simulink model "Simulink_Model_by_NV_PATEL"  (R2022a)
settings: Solver=VariableStepAuto  StartTime=0.0  StopTime=15  FixedStep=0.01  RelTol=1e-3
values from neighbouring files (symbols this model uses):
  direct_transmission_matrix = 0    [state_space_and_other_parameters.m]
  input_matrix = [0; 1/(m*l^2)]    [state_space_and_other_parameters.m]
  output_matrix = [1 0]    [state_space_and_other_parameters.m]
  Q = 1e-3    (= 0.001)    [state_space_and_other_parameters.m]
  R = 1e-4    (= 0.0001)    [state_space_and_other_parameters.m]
  system_matrix = [0 1; -g/l 0]    [state_space_and_other_parameters.m]
  Ts = 0.01    [state_space_and_other_parameters.m]
undefined symbols (not defined in the file or in its folder): Continuous, Time
libraries: simulink x2, ctrlSharedLib x1, Meldas_Library x1
settings Model: Creator=mulusoy  LastModifiedBy=jamesbond
settings SolverCC: AlgebraicLoopSolver=TrustRegion
settings DataIOCC: ReturnWorkspaceOutputs=off
settings OptimizationCC: DefaultParameterBehavior=Inlined  PassReuseOutputArgsAs=Individual arguments  EfficientTunableParamExpr=on
settings DebuggingCC: ParameterTunabilityLossMsg=error  UnconnectedInputMsg=warning  UnconnectedOutputMsg=warning  UnconnectedLineMsg=warning  SFMachineParentedDataDiag=warning  ArithmeticOperatorsInVariantConditions=warning
settings SFSimCC: SimUseLocalCustomCode=off  MATLABDynamicMemAlloc=off  CustomCodeUndefinedFunction=UseInterfaceOnly
settings RTWCC: SystemTargetFile=ert.tlc  TemplateMakefile=ert_default_tmf  GenerateReport=on  RTWUseLocalCustomCode=off  IncludeHyperlinkInReport=on  LaunchReport=on  GenerateTraceInfo=on  GenerateTraceReport=on  GenerateTraceReportSl=on  GenerateTraceReportSf=on  GenerateTraceReportEml=on  CheckMdlBeforeBuild=Warning
settings CodeAppCC: GenerateComments=off  IgnoreCustomStorageClasses=off  SimulinkBlockComments=off
settings ERTTargetCC: TargetLangStandard=C99 (ISO)  GenerateSampleERTMain=on  InlinedParameterPlacement=NonHierarchical  ERTCustomFileTemplate=example_file_process.tlc
settings SimscapeCC: SimscapeNormalizeSystem=off
settings ExplorerConfigSet: InternalSimMechanicsExplorerSettings="<ExplorerConfiguration><canonicalview>default</canonicalview><AnimationSetting><BasePlaybackSpeed>1.0</BasePlaybackSpeed><PlaybackSpeedFactor>1.0</PlaybackSpeedFactor></AnimationSetting><TilePanel><TileInfo><Tiles Columns=\"1\" Count=\"1\" Rows=\"1\"><Column Weight=\"1\"/><Row Weight=\"1\"/><Tile Height=\"1\" Width=\"1\" X=\"0\" Y=\"0\"/></Tiles></TileInfo><SceneInfo><SceneViewer><BGColor><R>0.60000002384185791</R><G>0.60000002384185791</G><B>0.60000002384185791</B></BGColor><Camera><DoPerspective>off</DoPerspective><Position><X>0.00439803475464691299</X><Y>-1.26266336441040039</Y><Z>0.0045894655792633049</Z></Position><Center><X>0.00439803475464691299</X><Y>-0.262663364410400391</Y><Z>0.0045894655792633049</Z></Center><Up><X>0</X><Y>-0</Y><Z>1</Z></Up><ViewLimDist>1</ViewLimDist><YLim>0.0755349543253689276</YLim><XLim>0.125636620232322499</XLim></Camera></SceneViewer></SceneInfo></TilePanel><MechEditorPanel><Cameras/><GfxPanelCameraMap/><VideoCreator><PlaybackSpeedRatio>1.0</PlaybackSpeedRatio><FrameRate>30</FrameRate><VideoFormat>Motion JPEG AVI</VideoFormat><FrameSize>auto</FrameSize></VideoCreator></MechEditorPanel></ExplorerConfiguration>"

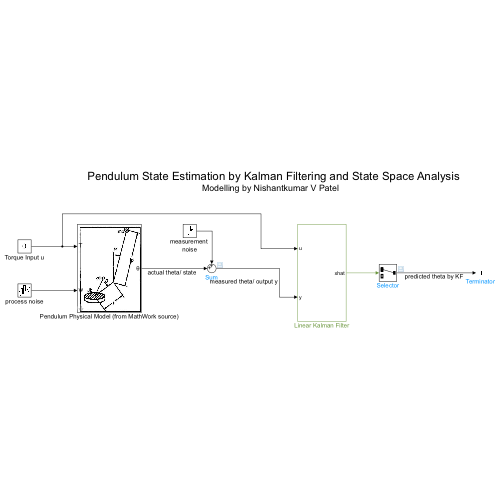
[thumbnail: Simulink's stored preview of the top-level diagram]
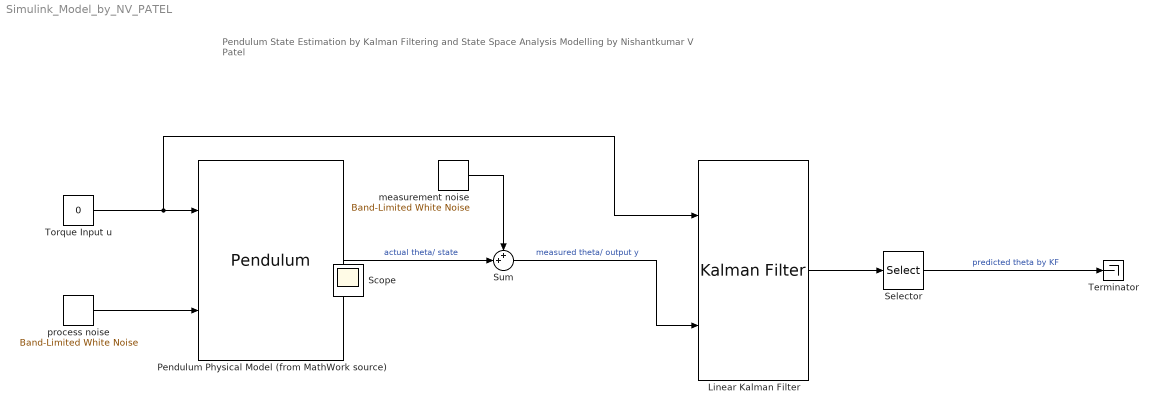
== system Simulink_Model_by_NV_PATEL ==
  note: Pendulum State Estimation by Kalman Filtering and State Space Analysis
      | Modelling by Nishantkumar V Patel
  Linear Kalman Filter : ctrlSharedLib/Kalman Filter  TimeDomain=Continuous-Time  UseCurrentEstimator=on  ModelSource=Individual A, B, C, D matrices  ModelSourceVariable=ss(0.95,1,1,0,1)  A=system_matrix  B=input_matrix  C=output_matrix  D=direct_transmission_matrix  NumberOfStates=1  NumberOfInputs=1  NumberOfOutputs=1  InitialEstimateSource=Dialog  X0=[pi/16 0]  P0=10  UseK=off  UseGH=off  NumberOfProcessNoiseInputs=1  G=1  TimeInvariantG=on  H=0  TimeInvariantH=on  Q=diag([0,Q])  TimeInvariantQ=on  R=R  TimeInvariantR=on  N=0  TimeInvariantN=on  AddInputPort=on  AddEnablePort=off  OutputEstimatedY=off  OutputP=off  Ts=0.01
  Pendulum Physical Model (from MathWork source) : Meldas_Library/Pendulum  theta_0=pi/4  theta_dot_0=0
  Selector : Selector  InputPortWidth=2  IndexOptions=Index vector (dialog)  Indices=1  OutputSizes=1
  Sum : Sum  Inputs=++|
  Terminator : Terminator
  Torque Input u : Constant  Value=0
  measurement noise : simulink/Sources/Band-Limited White Noise  Cov=R*Ts  Ts=Ts  seed=[12347]
  process noise : simulink/Sources/Band-Limited White Noise  Cov=Q*Ts  Ts=Ts  seed=[23341]
  Scope : Scope
  wires:
  Pendulum Physical Model (from MathWork source)/1 -> Sum/2  "actual theta/ state"
  measurement noise/1 -> Sum/1
  Sum/1 -> Linear Kalman Filter/2  "measured theta/ output y"
  Linear Kalman Filter/1 -> Selector/1
  Selector/1 -> Terminator/1  "predicted theta by KF"
  Torque Input u/1 -> Pendulum Physical Model (from MathWork source)/1, Linear Kalman Filter/1
  process noise/1 -> Pendulum Physical Model (from MathWork source)/2
